simulink model "EMG_FES2_calib"  (R2014a)
settings: Solver=FixedStepDiscrete  StartTime=0.0  StopTime=50  FixedStep=1/aFES.Fs  RelTol=1e-3
InitFcn:
  | if ~exist('aFES','var')
  |   load('afes_param')
  | 
  |    aFES.Fs=1000;
  |    if (~isfield(aFES,'stimCurr'))
  |        aFES.stimCurr=[15,15];
  |    end
  |    aFES.stimFreq=25;
  |    aFES.hand='left';
  | 
  |    %set run number
  |    if (isfield(aFES,'runNum'))
  |          aFES.runNum=aFES.runNum+1;
  |    else
  |          aFES.runNum=1;
  |    end
  | 
  |    %Bias
  |    aFES.wristPosZeroBias=1.8; %e.g: goniometer reading at zeros flexion and extension
  | 
  |    %Set the upper and lower safty limit of the sensor
  |    sensorUpperSafety1=aFES.activeSensorMax+(aFES.activeSensorMax-aFES.activeSensorMin)/4 ;
  |    sensorLowerSafety1=aFES.activeSensorMin-(aFES.activeSensorMax-aFES.activeSensorMin)/4 ;
  | 
  | 
  |    %% Feedback
  |    aFES=emgfes_feedback(aFES,0,0);
  |    aFES.doubleThresh=[0.2,0.4];%Ambrosini double threshold
  | 
  |    %% FIlters
  |    [EMG_bandpass_b,EMG_bandpass_a]=butter(5,2*[40,400]/aFES.Fs);
  | 
  |    %% Tracing
  |    aFES.tracing.reflectFeedback =-1;% {1,-1} e.g if the -1, gonirmeter signal will be multiplied by -1.
  |    aFES.tracing.MaxHeightFactor=1;%when >1 scales down the max traceable height. When < 1, scales up the max traceable hieght.
  |    [~,trap_y]=trapezoid4trace();%get the trapezium to be traced
  |    n_z=5;
  |    zero_pad=zeros(n_z*aFES.Fs,1);
  | 
  |    trap_yt=[[0:1/aFES.Fs:((((n_z*aFES.Fs)+2*length(trap_y))/aFES.Fs))-(1/aFES.Fs)]', [zero_pad;trap_y;-trap_y]]; %add time to the trap
  | 
  | end
StopFcn:
  | %save the calibration data but don't apply it
  | aFES.temp.passiveSensorMin=calib1_passiveSensorMin;
  | aFES.temp.passiveSensorMax=calib1_passiveSensorMax;
  | 
  | clear calib1_passiveSensorMin calib1_passiveSensorMax;
  | 
  | %save(['data/afes_data_run',mat2str(aFES.runNum),'.mat'],'aFES','pw_applied','rawProcSignal');
  | save(aFES.fn,'aFES','pw_applied','rawProcSignal');
  | disp('Passive Calibration data is saved');
  | 
  | disp('Passive Calibration data is updated but not applied. ');
  | disp('To apply it run: aFES.passiveSensorMin=aFES.temp.passiveSensorMin;  aFES.passiveSensorMax=aFES.temp.passiveSensorMax; ');
values from neighbouring files (symbols this model uses):
  trap_y = y'    [trapezoid4trace.m]
undefined symbols (not defined in the file or in its folder): analoginput, EMG_bandpass_a, EMG_bandpass_b, emgfes_feedback
libraries: dspmtrx3 x4, dspswit3 x3, simulink x2, dspinverses x2, daqlib x1, ScienceStimHasomed_Lib x1
settings Model: Creator=bethel.osuagwu  LastModifiedBy=bethel.osuagwu

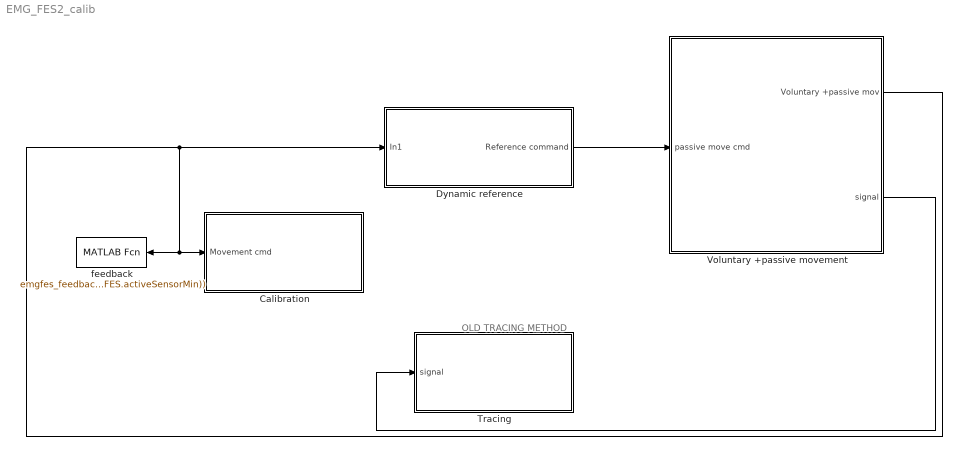
== system EMG_FES2_calib ==
  note: OLD TRACING METHOD
  Calibration : Subsystem
  Dynamic reference : Subsystem
  Tracing : Subsystem
  Voluntary +passive movement : Subsystem
  feedback : MATLABFcn  MATLABFcn=emgfes_feedback(aFES,(u'-aFES.activeSensorMin)./(aFES.activeSensorMax-aFES.activeSensorMin))  OutputDimensions=0
  wires:
  Dynamic reference/1(Reference command) -> Voluntary +passive movement/1(passive move cmd)
  Voluntary +passive movement/1(Voluntary +passive mov) -> feedback/1, Calibration/1(Movement cmd), Dynamic reference/1(In1)
  Voluntary +passive movement/2(signal) -> Tracing/1(signal)

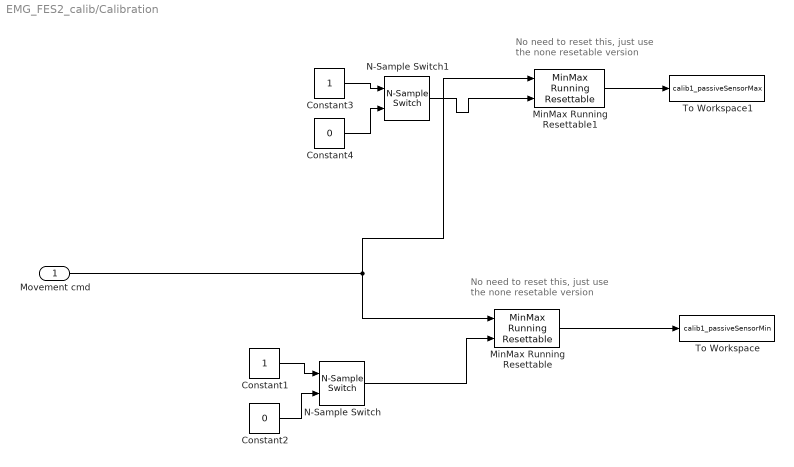
== system EMG_FES2_calib/Calibration ==
  note: No need to reset this, just use
      |  the none resetable version
  note: No need to reset this, just use
      |  the none resetable version
  Movement cmd : Inport
  Constant1 : Constant
  Constant2 : Constant  Value=0
  Constant3 : Constant
  Constant4 : Constant  Value=0
  MinMax Running Resettable : simulink/Math Operations/MinMax Running Resettable  Function=min  vinit=inf
  MinMax Running Resettable1 : simulink/Math Operations/MinMax Running Resettable  Function=max  vinit=-inf
  N-Sample Switch : dspswit3/N-Sample Switch  N=10000  reset=off  TriggerType=Rising edge  Ts=-1
  N-Sample Switch1 : dspswit3/N-Sample Switch  N=10000  reset=off  TriggerType=Rising edge  Ts=-1
  To Workspace : ToWorkspace  VariableName=calib1_passiveSensorMin  SampleTime=-1
      settings: MaxDataPoints=1
  To Workspace1 : ToWorkspace  VariableName=calib1_passiveSensorMax  SampleTime=-1
      settings: MaxDataPoints=1
  wires:
  N-Sample Switch1/1 -> MinMax Running Resettable1/2
  Constant1/1 -> N-Sample Switch/1
  MinMax Running Resettable1/1 -> To Workspace1/1
  MinMax Running Resettable/1 -> To Workspace/1
  N-Sample Switch/1 -> MinMax Running Resettable/2
  Constant2/1 -> N-Sample Switch/2
  Constant3/1 -> N-Sample Switch1/1
  Constant4/1 -> N-Sample Switch1/2
  Movement cmd/1 -> MinMax Running Resettable1/1, MinMax Running Resettable/1

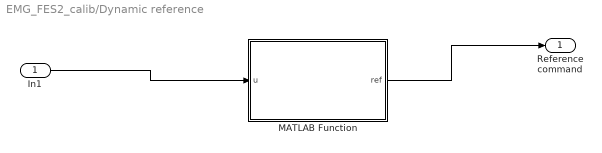
== system EMG_FES2_calib/Dynamic reference ==
  In1 : Inport
  MATLAB Function : MATLAB Function  TreatAsAtomicUnit=on
  Reference command : Outport
  wires:
  MATLAB Function/1(ref) -> Reference command/1
  In1/1 -> MATLAB Function/1(u)

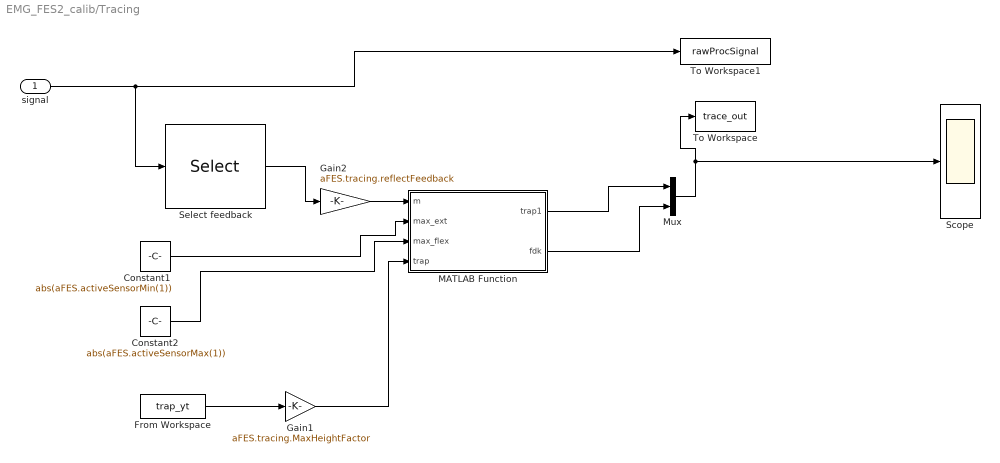
== system EMG_FES2_calib/Tracing ==
  signal : Inport
  Constant1 : Constant  Value=abs(aFES.activeSensorMin(1))
  Constant2 : Constant  Value=abs(aFES.activeSensorMax(1))
  From Workspace : FromWorkspace  VariableName=trap_yt  SampleTime=1/aFES.Fs  OutputAfterFinalValue=Setting to zero
  Gain1 : Gain  Gain=aFES.tracing.MaxHeightFactor
  Gain2 : Gain  Gain=aFES.tracing.reflectFeedback
  MATLAB Function : MATLAB Function  TreatAsAtomicUnit=on
  Mux : Mux  Inputs=2
  Scope : Scope
      settings: YMin=-3.5  YMax=1  SaveName=ScopeData2
  Select feedback : Selector  InputPortWidth=9  Indices=[7]
  To Workspace : ToWorkspace  VariableName=trace_out  SampleTime=-1
  To Workspace1 : ToWorkspace  VariableName=rawProcSignal  SampleTime=-1
  wires:
  MATLAB Function/1(trap1) -> Mux/1
  Mux/1 -> To Workspace/1, Scope/1
  Gain1/1 -> MATLAB Function/4(trap)
  Constant1/1 -> MATLAB Function/2(max_ext)
  Constant2/1 -> MATLAB Function/3(max_flex)
  signal/1 -> Select feedback/1, To Workspace1/1
  From Workspace/1 -> Gain1/1
  MATLAB Function/2(fdk) -> Mux/2
  Select feedback/1 -> Gain2/1
  Gain2/1 -> MATLAB Function/1(m)

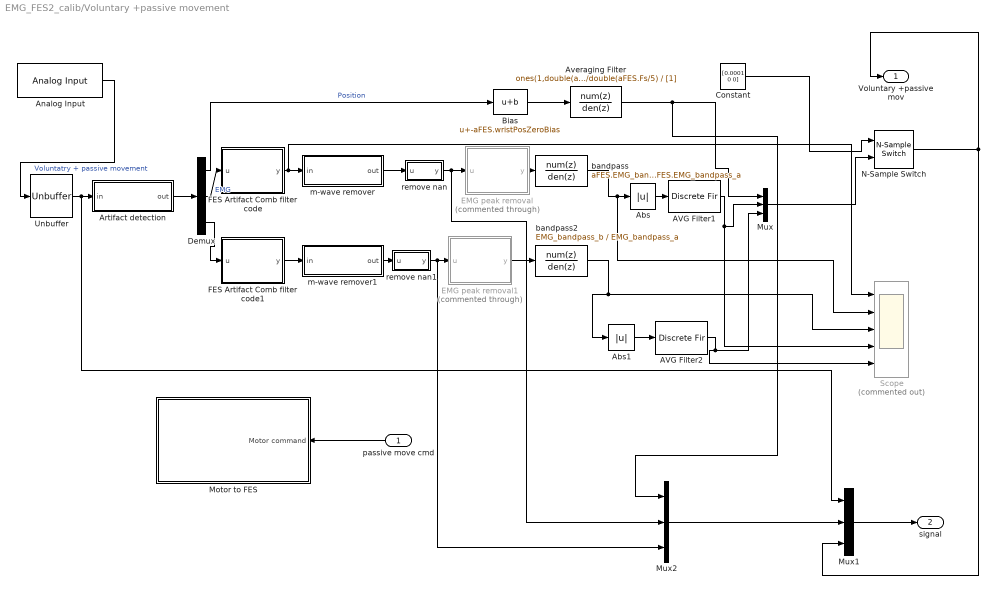
== system EMG_FES2_calib/Voluntary +passive movement ==
  passive move cmd : Inport
  " AVG Filter1" : DiscreteFir  Coefficients=ones(1,1000)/1000
  " AVG Filter2" : DiscreteFir  Coefficients=ones(1,1000)/1000
  Abs : Abs
  Abs1 : Abs
  Analog Input : daqlib/Analog Input  AcqMode=0  DeviceMenu=nidaq Dev1 (USB-6341 (BNC))  Device=nidaq Dev1 (USB-6341 (BNC))  ObjConstructor=analoginput('nidaq','Dev1')  SampleRate=1000  ActualRate=1000  SamplesPerFrame=2  InputType=Differential  NChannelsSelected=3  Channels=1$0$$2$#1$1$$2$#1$2$$2$#0$3$$1$#0$4$$1$#0$5$$1$#0$6$$1$#0$7$$1$#  NPorts=1 for all hardware channels  DataType=double
      settings: SignalType=Sample-based
  Artifact detection : Subsystem
  Averaging Filter : DiscreteFilter  Numerator=ones(1,double(aFES.Fs/5))/double(aFES.Fs/5)  Denominator=[1]
  Bias : Bias  Bias=-aFES.wristPosZeroBias
  Constant : Constant  Value=[0.0001 0 0]
  Demux : Demux  Outputs=3
  EMG peak removal : MATLAB Function  Commented=through  TreatAsAtomicUnit=on
  EMG peak removal1 : MATLAB Function  Commented=through  TreatAsAtomicUnit=on
  FES Artifact Comb filter code : MATLAB Function  TreatAsAtomicUnit=on
  FES Artifact Comb filter code1 : MATLAB Function  TreatAsAtomicUnit=on
  Motor to FES : Subsystem
  Mux : Mux  Inputs=3
  Mux1 : Mux  Inputs=3
  Mux2 : Mux  Inputs=3
  N-Sample Switch : dspswit3/N-Sample Switch  N=10  reset=off  TriggerType=Rising edge  Ts=-1
  Scope : Scope  Commented=on  NumInputPorts=5
      settings: YMin=-2.5~-0.5~-0.3~0~0  YMax=2.5~0.4~0.4~0.025~0.035
  Unbuffer : Unbuffer  SampleBasedProcessing=Same as frame based
  bandpass : DiscreteFilter  Numerator=aFES.EMG_bandpass_b  Denominator=aFES.EMG_bandpass_a
  bandpass2 : DiscreteFilter  Numerator=EMG_bandpass_b  Denominator=EMG_bandpass_a
  m-wave remover : Subsystem
  m-wave remover1 : Subsystem
  remove nan : MATLAB Function  TreatAsAtomicUnit=on
  remove nan1 : MATLAB Function  TreatAsAtomicUnit=on
  Voluntary +passive mov : Outport
  signal : Outport  Port=2
  wires:
  Analog Input/1 -> Unbuffer/1  "Voluntatry + passive movement"
  Demux/1 -> Bias/1  "Position"
  Abs/1 -> " AVG Filter1"/1
  " AVG Filter1"/1 -> Scope/4, Mux/2
  passive move cmd/1 -> Motor to FES/1(Motor command)
  Demux/2 -> FES Artifact Comb filter code/1(u)  "EMG"
  Constant/1 -> N-Sample Switch/1
  N-Sample Switch/1 -> Mux1/3, Voluntary +passive mov/1
  Unbuffer/1 -> Mux1/1, Artifact detection/1(in)
  Bias/1 -> Averaging Filter/1
  Averaging Filter/1 -> Mux2/1, Mux/1
  Abs1/1 -> " AVG Filter2"/1
  " AVG Filter2"/1 -> Scope/5, Mux/3
  Demux/3 -> FES Artifact Comb filter code1/1(u)
  FES Artifact Comb filter code/1(y) -> Scope/1, m-wave remover/1(in)
  EMG peak removal1/1(y) -> bandpass2/1
  Mux/1 -> N-Sample Switch/2
  Artifact detection/1(out) -> Demux/1
  m-wave remover/1(out) -> remove nan/1(u)
  FES Artifact Comb filter code1/1(y) -> m-wave remover1/1(in)
  EMG peak removal/1(y) -> bandpass/1
  bandpass/1 -> Scope/2, Abs/1
  bandpass2/1 -> Abs1/1, Scope/3
  remove nan/1(y) -> Mux2/2, EMG peak removal/1(u)
  remove nan1/1(y) -> Mux2/3, EMG peak removal1/1(u)
  m-wave remover1/1(out) -> remove nan1/1(u)
  Mux1/1 -> signal/1
  Mux2/1 -> Mux1/2

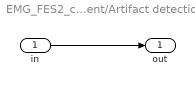
== system EMG_FES2_calib/Voluntary +passive movement/Artifact detection ==
  in : Inport
  out : Outport
  wires:
  in/1 -> out/1

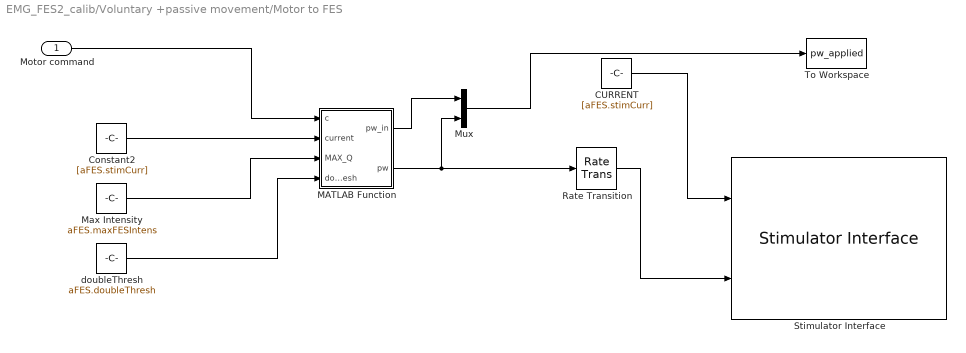
== system EMG_FES2_calib/Voluntary +passive movement/Motor to FES ==
  Motor command : Inport
  CURRENT : Constant  Value=[aFES.stimCurr]
  Constant2 : Constant  Value=[aFES.stimCurr]
  MATLAB Function : MATLAB Function  TreatAsAtomicUnit=on
  Max Intensity : Constant  Value=aFES.maxFESIntens
  Mux : Mux  Inputs=2
  Rate Transition : RateTransition
  Stimulator Interface : ScienceStimHasomed_Lib/Stimulator Interface  Ts=33/aFES.Fs  com_port=COM9  channelstim=[1,2]  tsone=round((1/aFES.stimFreq)*1000)  tstwo=5  channellf=[]  nfactor=[]  outflag=off  dtflag=off
  To Workspace : ToWorkspace  VariableName=pw_applied  SampleTime=-1
  doubleThresh : Constant  Value=aFES.doubleThresh
  wires:
  CURRENT/1 -> Stimulator Interface/1
  Motor command/1 -> MATLAB Function/1(c)
  MATLAB Function/2(pw) -> Mux/2, Rate Transition/1
  Rate Transition/1 -> Stimulator Interface/2
  Constant2/1 -> MATLAB Function/2(current)
  Max Intensity/1 -> MATLAB Function/3(MAX_Q)
  doubleThresh/1 -> MATLAB Function/4(doubleThresh)
  MATLAB Function/1(pw_in) -> Mux/1
  Mux/1 -> To Workspace/1

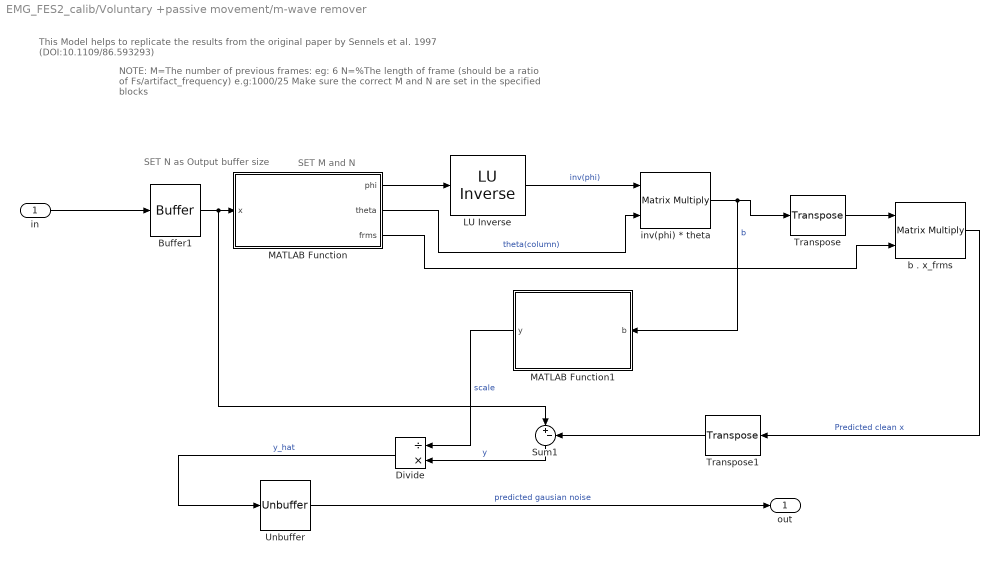
== system EMG_FES2_calib/Voluntary +passive movement/m-wave remover ==
  note: NOTE:
      | M=The number of previous frames: eg: 6
      | N=%The length of frame (should be a ratio of Fs/artifact_frequency) e.g:1000/25
      | Make sure the correct M and N are set in the specified blocks
  note: SET N as Output
      | buffer size
  note: SET M and N
  note: This Model helps to replicate the results from the original paper by Sennels et al. 1997 (DOI:10.1109/86.593293)
  in : Inport
  " LU Inverse" : dspinverses/ LU Inverse
  Buffer1 : Buffer  N=40  TreatMby1Signals=One channel
  Divide : Product  Inputs=/*
  MATLAB Function : MATLAB Function  TreatAsAtomicUnit=on
  MATLAB Function1 : MATLAB Function  TreatAsAtomicUnit=on
  Sum1 : Sum  Inputs=|+-
  Transpose : dspmtrx3/Transpose  Hermitian=off  overflowFlag=off
  Transpose1 : dspmtrx3/Transpose  Hermitian=off  overflowFlag=off
  Unbuffer : Unbuffer  SampleBasedProcessing=Same as frame based
  b . x_frms : Product  Multiplication=Matrix(*)
  inv(phi) * theta : Product  Multiplication=Matrix(*)
  out : Outport
  wires:
  Buffer1/1 -> Sum1/1, MATLAB Function/1(x)
  MATLAB Function/1(phi) -> " LU Inverse"/1
  MATLAB Function/2(theta) -> inv(phi) * theta/2  "theta(column)"
  " LU Inverse"/1 -> inv(phi) * theta/1  "inv(phi)"
  inv(phi) * theta/1 -> MATLAB Function1/1(b), Transpose/1  "b"
  Unbuffer/1 -> out/1  "predicted gausian noise"
  MATLAB Function/3(frms) -> b . x_frms/2
  Transpose/1 -> b . x_frms/1
  b . x_frms/1 -> Transpose1/1  "Predicted clean x"
  Transpose1/1 -> Sum1/2
  Sum1/1 -> Divide/2  "y"
  MATLAB Function1/1(y) -> Divide/1  "scale"
  Divide/1 -> Unbuffer/1  "y_hat"
  in/1 -> Buffer1/1

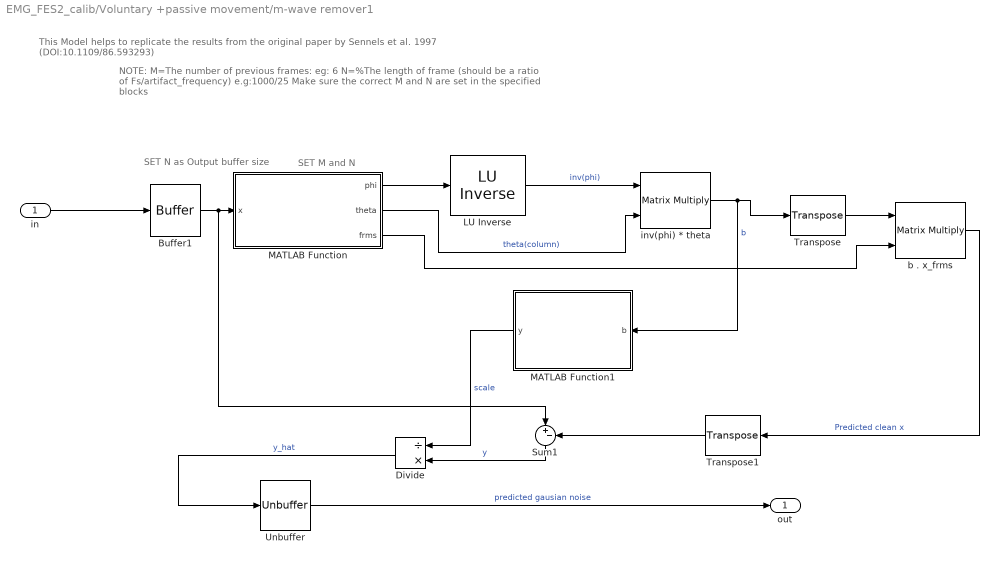
== system EMG_FES2_calib/Voluntary +passive movement/m-wave remover1 ==
  note: NOTE:
      | M=The number of previous frames: eg: 6
      | N=%The length of frame (should be a ratio of Fs/artifact_frequency) e.g:1000/25
      | Make sure the correct M and N are set in the specified blocks
  note: SET N as Output
      | buffer size
  note: SET M and N
  note: This Model helps to replicate the results from the original paper by Sennels et al. 1997 (DOI:10.1109/86.593293)
  in : Inport
  " LU Inverse" : dspinverses/ LU Inverse
  Buffer1 : Buffer  N=80  TreatMby1Signals=One channel
  Divide : Product  Inputs=/*
  MATLAB Function : MATLAB Function  TreatAsAtomicUnit=on
  MATLAB Function1 : MATLAB Function  TreatAsAtomicUnit=on
  Sum1 : Sum  Inputs=|+-
  Transpose : dspmtrx3/Transpose  Hermitian=off  overflowFlag=off
  Transpose1 : dspmtrx3/Transpose  Hermitian=off  overflowFlag=off
  Unbuffer : Unbuffer  SampleBasedProcessing=Same as frame based
  b . x_frms : Product  Multiplication=Matrix(*)
  inv(phi) * theta : Product  Multiplication=Matrix(*)
  out : Outport
  wires:
  Buffer1/1 -> Sum1/1, MATLAB Function/1(x)
  MATLAB Function/1(phi) -> " LU Inverse"/1
  MATLAB Function/2(theta) -> inv(phi) * theta/2  "theta(column)"
  " LU Inverse"/1 -> inv(phi) * theta/1  "inv(phi)"
  inv(phi) * theta/1 -> MATLAB Function1/1(b), Transpose/1  "b"
  Unbuffer/1 -> out/1  "predicted gausian noise"
  MATLAB Function/3(frms) -> b . x_frms/2
  Transpose/1 -> b . x_frms/1
  b . x_frms/1 -> Transpose1/1  "Predicted clean x"
  Transpose1/1 -> Sum1/2
  Sum1/1 -> Divide/2  "y"
  MATLAB Function1/1(y) -> Divide/1  "scale"
  Divide/1 -> Unbuffer/1  "y_hat"
  in/1 -> Buffer1/1

== matlab function EMG_FES2_calib/Dynamic reference/MATLAB Function ==
  data: ref output; u input
function ref   = fcn(u)
%#codegen
persistent ts ts_c ref_mem;
ref_delta=0.0013;
Fs=1000;
if(isempty(ts))
    ts=0;
    ts_c=0;
    ref_mem=[0;0];
end
ts=ts+1;



ref=ref_mem;
if(ts>Fs*4)
    ts_c=ts_c+1;
    if(ts_c<Fs*4)
        ref(1)=ref(1)+ref_delta;
        ref(2)=0;
    elseif ts_c<Fs*8
        ref(2)=ref(2)+ref_delta;
        ref(1)=0;
    elseif ts_c>=Fs*8
        ref(1)=0;
        ref(2)=0;
        ts_c=0;
    end
end
ref_mem=ref;

== matlab function EMG_FES2_calib/Voluntary +passive movement/FES Artifact Comb filter code ==
  data: u input; y output
function y  = fcn(u)
%#codegen

persistent u_mem;
fes_freq=25;%FES frequency
Fs=1000;%EMG/data samplerate
K=40;%round(Fs/fes_freq); %Comb filter order = (1/fes_freq)*Fs
a=-1;%{-1 to 0}
if isempty(u_mem)
    u_mem=zeros(K,1);
end





%% Comb filtering
% Forward comb
y=u+ a*u_mem(1);



u_mem(1:end-1)=u_mem(2:end);
u_mem(end)=u;



end





%

== matlab function EMG_FES2_calib/Voluntary +passive movement/Motor to FES/MATLAB Function ==
  data: pw_in output; c input; current input; pw output; MAX_Q input; doubleThresh input
function [pw_in,pw] = fcn(c,current,MAX_Q,doubleThresh)
%#codegen
% c is the controller output
% dcdt is the derivative of c
%MAX_Q= eg.5000;%maxmum intensity =current x pulsewidth
persistent  FES_ON pw_smooth;

pMax=300;
if isempty(pw_smooth)
    %c_mem=zeros(30,2);
    FES_ON=[0;0];
    pw_smooth=[0;0];
end


%% (Module) Avoid spikes in Stimulation
% if false
% c(dcdt>0.5)=median(c_mem);
% %upadte memory of controller output
%  c_mem(1:end-1,:)=c_mem(2:end,:);
%  c_mem(end,:)=c;
% end

%compute pulsewidth
if(doubleThresh(2))
    pw=[0;0];
    for chni=1:2
        if FES_ON(chni)
            if c(chni)<doubleThresh(1)
                pw(chni)=0;
                FES_ON(chni)=0;
            else
                pw(chni)=200+c(chni).*30;
                FES_ON(chni)=1;
            end
        else %it is currently off
            if c(chni)>doubleThresh(2)
                pw(chni)=200+c(chni).*30;
                FES_ON(chni)=1;
            else
                pw(chni)=0;
                FES_ON(chni)=0;
            end
        end
    end
    
else
    pw=(c).*pMax;
    pw(pw<0)=0;
    %pw(pw>50)=pw(pw>50)+10;%add a bias
    pw(pw<50)=0;
end

%% Limit max Intensity of FES
q=current.*pw;
q_=q>MAX_Q;
for nq=1:length(q_)
    if q_(nq)
        pw(nq)=MAX_Q/current(nq);
        'Motor to FES: limits [ch,pulsewidth_limit]'
        [nq pw(nq)]
    end
end

%% The estimated pw is essentially our input pw
pw_in=pw;% If no further modification below, then pw_in==pw


%% (Module)Controller output based change in stimulation for opposing movement assistance



%% (Module)Error based change in stimulation for opposing movement assistance


%% (Module) Smoothness controller for pw
pw_step=0.2;%(TODO: should be a function of max pw and samplerate)allowed positive step chnage per sample
pw=abs(pw_smooth+sign(pw-pw_smooth)*pw_step); %the abs here is fine as far as the step size is small(e.g <5)
%pw(pw<pw_step)=0;NOTE open this 
pw_smooth=pw;
%-----------------------------

== matlab function EMG_FES2_calib/Voluntary +passive movement/m-wave remover/MATLAB Function ==
  data: x input; phi output double; theta output; frms output
function [phi,theta,frms] = fcn(x)
%#codegen
persistent t_sample phi_mem  frms_mem ;

%General param
M=6; %The number of previous frames 
N=40; %The length of frame (should be a ratio of Fs/artifact_frequency)

% Performance parameter
freshPhi =1;% when =1:recompute phi(covariance matix) all the phi; when =0:update phi with only new values

if isempty(t_sample)
    t_sample=0;
    frms_mem=zeros(M,N);
    
    phi_mem=zeros(M,M);
end
t_sample=t_sample+1;

%make x a row vector
x=x';


%% compute phi
frms=frms_mem;
%equ 7 and 8
if(freshPhi)
    % compute phi fresh all the time
    phi=(frms*frms');
else
    %we can compute only the required column (first) and row (first)of phi
    %matrix and push the new values into phi
    phi_mem(2:end,2:end)=phi_mem(1:end-1,1:end-1);
    phi_mem(1,:)=frms(1,:)*frms';
    phi_mem(:,1)=phi_mem(1,:)';
    %phi-phi_mem
    phi=phi_mem;
end


%% compute theta
theta=(x*frms')';
%t_sample
%if t_sample==15
%    y=4;
%end


%% update frame
frms_mem(2:end,:)=frms_mem(1:end-1,:);
frms_mem(1,:)=x;

== matlab function EMG_FES2_calib/Voluntary +passive movement/FES Artifact Comb filter code1 ==
  data: u input; y output
function y  = fcn(u)
%#codegen

persistent u_mem;
fes_freq=25;%FES frequency
Fs=1000;%EMG/data samplerate
K=40;%round(Fs/fes_freq); %Comb filter order = (1/fes_freq)*Fs
a=-1;%{-1 to 0}
if isempty(u_mem)
    u_mem=zeros(K,1);
end





%% Comb filtering
% Forward comb
y=u+ a*u_mem(1);



u_mem(1:end-1)=u_mem(2:end);
u_mem(end)=u;
end





%

== matlab function EMG_FES2_calib/Voluntary +passive movement/EMG peak removal1 ==
  data: u input; y output
function y  = fcn(u)
%#codegen
%peak removal
peak_thresh=0.5;
dmdt_thresh=0.3;
blocking_win=50;
persistent u_mem t_;
if isempty(u_mem)
    u_mem=zeros(1000,1);
    t_=0;
end

if (dmdt_thresh<abs(u)-abs(u_mem(end))&& t_==0)%if the change in value to too large  then block with no stats
    t_=1;
else   
    if((abs(u)>peak_thresh || dmdt_thresh<abs(u)-abs(u_mem(end))) && t_==0) %detect high amplitude,peak, and start blocking
        if(abs(u)>std(u_mem))
            t_=1;
        end
    end

    
end


if t_
    u=0;%block
   t_=t_+1;
end
if(t_==blocking_win) %stop blocking after n samples
    t_=0; 
end

u_mem(1:end-1)=u_mem(2:end);
u_mem(end)=u;
y=u;
end





%

== matlab function EMG_FES2_calib/Voluntary +passive movement/EMG peak removal ==
  data: u input; y output
function y  = fcn(u)
%#codegen
%peak removal
peak_thresh=0.5;
dmdt_thresh=0.3;
blocking_win=50;
persistent u_mem t_;
if isempty(u_mem)
    u_mem=zeros(1000,1);
    t_=0;
end

if (dmdt_thresh<abs(u)-abs(u_mem(end))&& t_==0)%if the change in value to too large  then block with no stats
    t_=1;
else   
    if((abs(u)>peak_thresh || dmdt_thresh<abs(u)-abs(u_mem(end))) && t_==0) %detect high amplitude,peak, and start blocking
        if(abs(u)>std(u_mem))
            t_=1;
        end
    end

    
end


if t_
    u=0;%block
   t_=t_+1;
end
if(t_==blocking_win) %stop blocking after n samples
    t_=0; 
end

u_mem(1:end-1)=u_mem(2:end);
u_mem(end)=u;
y=u;
end





%

== matlab function EMG_FES2_calib/Voluntary +passive movement/remove nan ==
  data: u input; y output
function y  = fcn(u)
%#codegen

y=u;
if isnan(y)
    y=0;
end





%

== matlab function EMG_FES2_calib/Voluntary +passive movement/remove nan1 ==
  data: u input; y output
function y  = fcn(u)
%#codegen

y=u;
if isnan(y)
    y=0;
end





%

== matlab function EMG_FES2_calib/Voluntary +passive movement/m-wave remover/MATLAB Function1 ==
  data: b input; y output
function y = fcn(b)
%#codegen


y = sqrt(1+sum(b.^2));
%       OR
%y = (1+sum(b));%approximated for speed

== matlab function EMG_FES2_calib/Voluntary +passive movement/m-wave remover1/MATLAB Function ==
  data: x input; phi output double; theta output; frms output
function [phi,theta,frms] = fcn(x)
%#codegen
persistent t_sample phi_mem  frms_mem ;

%General param
M=6; %The number of previous frames 
N=80; %The length of frame (should be a ratio of Fs/artifact_frequency)

% Performance parameter
freshPhi =1;% when =1:recompute phi(covariance matix) all the phi; when =0:update phi with only new values

if isempty(t_sample)
    t_sample=0;
    frms_mem=zeros(M,N);
    
    phi_mem=zeros(M,M);
end
t_sample=t_sample+1;

%make x a row vector
x=x';


%% compute phi
frms=frms_mem;
%equ 7 and 8
if(freshPhi)
    % compute phi fresh all the time
    phi=(frms*frms');
else
    %we can compute only the required column (first) and row (first)of phi
    %matrix and push the new values into phi
    phi_mem(2:end,2:end)=phi_mem(1:end-1,1:end-1);
    phi_mem(1,:)=frms(1,:)*frms';
    phi_mem(:,1)=phi_mem(1,:)';
    %phi-phi_mem
    phi=phi_mem;
end


%% compute theta
theta=(x*frms')';
%t_sample
%if t_sample==15
%    y=4;
%end


%% update frame
frms_mem(2:end,:)=frms_mem(1:end-1,:);
frms_mem(1,:)=x;

== matlab function EMG_FES2_calib/Voluntary +passive movement/m-wave remover1/MATLAB Function1 ==
  data: b input; y output
function y = fcn(b)
%#codegen


y = sqrt(1+sum(b.^2));
%       OR
%y = (1+sum(b));%approximated for speed

== matlab function EMG_FES2_calib/Tracing/MATLAB Function ==
  data: m input; max_ext input; max_flex input; trap input; trap1 output; fdk output
function [trap1,fdk]    = fcn(m,max_ext,max_flex,trap)
%#codegen
%coder.extrinsic('plot','hold');
% persistent ts;
% if isempty(ts)
%     ts=0;
%     %m_mem=zeros(10*1000,1);
% end
%m_mem(1:end-1)=m_mem(2:end);
%m_mem(end)=m(1);

%scale extension
if(m(1)>0)
    m(1)=m(1)/max_ext;
elseif m(1)<0
    m(1)=m(1)/max_flex;
end
    
%ts=ts+1;
 trap1=trap;
 
 fdk=m(1);
 
%stopSingnal=0;
%  if(ts==length(trap))
%      stopSingnal=1;
%  end
